simulink model "mdl_collective_dynamics"  (R2021b)
settings: Solver=ode4  StartTime=0.0  StopTime=110  FixedStep=1e-3  RelTol=1e-3
values from neighbouring files (symbols this model uses):
  A = [0 1 1 1 1 1 1 1 1 1 1 1 ... (16384 elements, 128x128)]    [case_positive_means.mat]    (also in export_fig.m = {A}; fcn_general_dynamics.m = diag(A).*eye(numel(x)); newResultsMoreRobots_3.mat; newResultsMoreRobots_4.mat)
  c0 = 100    [fcn_general_dynamics.m]    (also in scrpt_collective_learning_dynamics.m; scrpt_learning_paradigms.m; scrpt_learning_paradigms_case_study_results.m; scrpt_learning_paradigms_case_study_statistics.m)
  N = length(tspan)    [ode4.m]    (also in ode4_sat.m; scrpt_collective_learning_dynamics.m = 3; scrpt_learning_paradigms.m = 3; scrpt_learning_paradigms_case_study_results.m = 3)
  tau = -log(threshold)*ones(N,1)    [scrpt_collective_learning_dynamics.m]    (also in scrpt_learning_paradigms.m = -log(epsilon)*ones(m,1); scrpt_learning_paradigms_case_study_results.m = -log(epsilon)*ones(m,1); scrpt_learning_paradigms_case_study_statistics.m = -log(epsilon)*ones(numberOfRobots,1); scrpt_learning_paradigms_case_study_varying_parameters.m = -log(parameters.knowledgeLowerBound)*ones(numberOfRobots,1))
settings Model: Creator=diaz  LastModifiedBy=diaz

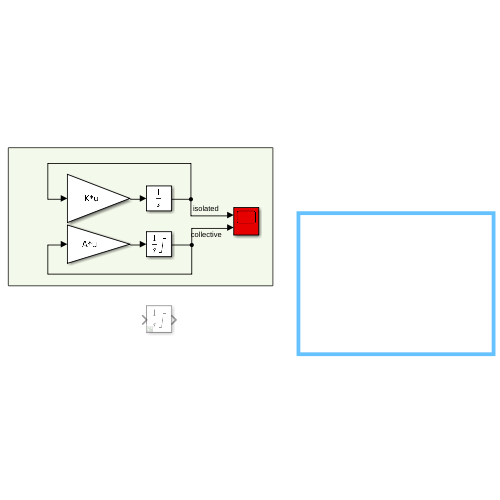
[thumbnail: Simulink's stored preview of the top-level diagram]
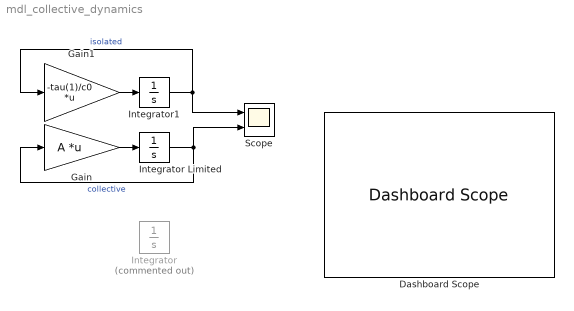
== system mdl_collective_dynamics ==
  Dashboard Scope : DashboardScope  Ymin=-0.1  Ymax=1.1
  Gain : Gain  Gain=A  Multiplication=Matrix(K*u)
  Gain1 : Gain  Gain=-tau(1)/c0  Multiplication=Matrix(K*u)
  Integrator : Integrator  Commented=on  InitialCondition=ones(N,1)  LimitOutput=on  UpperSaturationLimit=1  LowerSaturationLimit=0  WrappedStateUpperValue=1  WrappedStateLowerValue=0
  Integrator Limited : Integrator  InitialCondition=ones(N,1)  LimitOutput=on  UpperSaturationLimit=1  LowerSaturationLimit=0
  Integrator1 : Integrator  InitialCondition=1  LowerSaturationLimit=0
  Scope : Scope  NumInputPorts=2
  wires:
  Gain/1 -> Integrator Limited/1
  Integrator Limited/1 -> Gain/1, Scope/2  "collective"
  Gain1/1 -> Integrator1/1
  Integrator1/1 -> Scope/1, Gain1/1  "isolated"
